simulink model "Question_1"  (R2024b)
settings: Solver=VariableStepAuto  StartTime=0.0  StopTime=10.0  RelTol=1e-3
model workspace (MAT data in the model file):
  M1 = 20
  M2 = 20
  b1 = 6
  b2 = 10
  k = 5
settings Model: Creator=Sagar  LastModifiedBy=Sagar

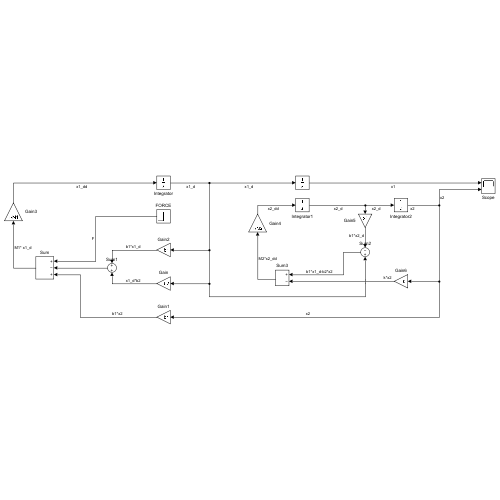
[thumbnail: Simulink's stored preview of the top-level diagram]
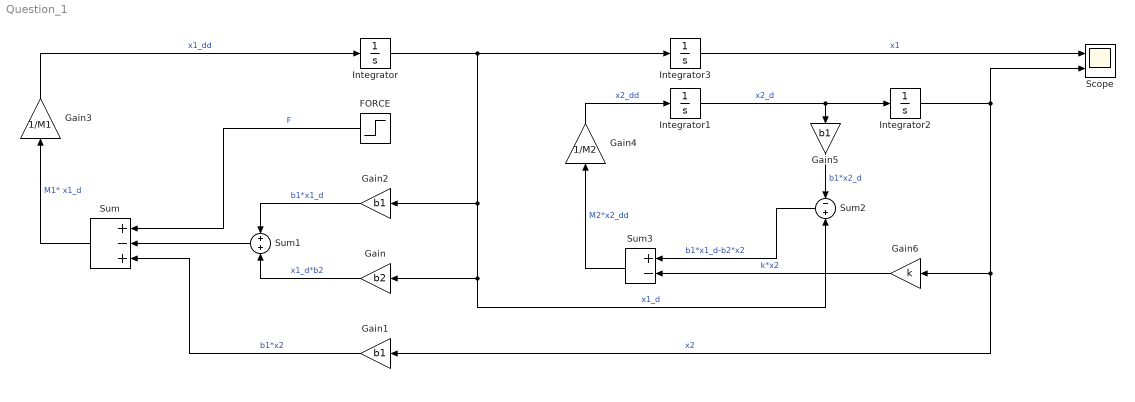
== system Question_1 ==
  FORCE : Step  SampleTime=0
  Gain : Gain  Gain=b2
  Gain1 : Gain  Gain=b1
  Gain2 : Gain  Gain=b1
  Gain3 : Gain  Gain=1/M1
  Gain4 : Gain  Gain=1/M2
  Gain5 : Gain  Gain=b1
  Gain6 : Gain  Gain=k
  Integrator{,1..3} (4 alike) : Integrator
  Scope : Scope  NumInputPorts=2
  Sum : Sum  Inputs=+-+
  Sum1 : Sum
  Sum2 : Sum  Inputs=-+
  Sum3 : Sum  Inputs=+-
  wires:
  Integrator/1 -> Integrator3/1, Gain2/1, Sum2/2, Gain/1  "x1_d"
  Gain3/1 -> Integrator/1  "x1_dd"
  Sum/1 -> Gain3/1  "M1* x1_d"
  Sum1/1 -> Sum/2
  Gain2/1 -> Sum1/1  "b1*x1_d"
  Gain/1 -> Sum1/2  "x1_d*b2"
  FORCE/1 -> Sum/1  "F"
  Gain1/1 -> Sum/3  "b1*x2"
  Gain4/1 -> Integrator1/1  "x2_dd"
  Integrator1/1 -> Integrator2/1, Gain5/1  "x2_d"
  Gain5/1 -> Sum2/1  "b1*x2_d"
  Integrator2/1 -> Scope/2, Gain6/1, Gain1/1  "x2"
  Gain6/1 -> Sum3/2  "k*x2"
  Sum3/1 -> Gain4/1  "M2*x2_dd"
  Sum2/1 -> Sum3/1  "b1*x1_d-b2*x2"
  Integrator3/1 -> Scope/1  "x1"
